simulink model "PubIfDecisionTOS_MDL"  (R2020b)
settings: configuration reference "DspaceConfig" (kept outside this file)
PostLoadFcn:
  | if any(exist('dsrtsu_mdlpostloadfcn', 'file') ~= 0), dsrtsu_mdlpostloadfcn('Execute', bdroot); end
InitFcn:
  | , if any(exist('dsmpb_private', 'file') ~= 0), dsmpb_private('dsmpb_mdlclblib', 'Init', bdroot); end,
undefined symbols (not defined in the file or in its folder): C_TOS_ACCEgoRAxletoFbumplength_m, C_TOS_ACCTargetFront_Flag, C_TOS_AEBJAPedObjDxThre_Val, C_TOS_AEBJAPedObjDyThre_Val, C_TOS_AEBJATargetSize_Val, C_TOS_AEBJAVehObjDxThre_Val, C_TOS_AEBJAVehObjDyThre_Val, C_TOS_AEBJuncPedTargetSize_Val, C_TOS_AEBLatObjDxThre_Val, C_TOS_AEBLatPedDyThre_Val, C_TOS_AEBLatTargetSize_Val, C_TOS_AEBLongTargetInEgoFront_Flag, C_TOS_axAbsGround_Parameter, C_TOS_CameraConfirmedFlag, C_TOS_CNsubjWidth, C_TOS_CurrentLaneCoreMinWidth_Val, C_TOS_CutInProb_Val_Zero, C_TOS_CutOutProb_Val_Zero, C_TOS_D2R_Val, C_TOS_DefaultValueObjectToCenterLine_dy, C_TOS_EgoCarWidth_Val, C_TOS_EgoDxRefPoint_m, C_TOS_EgoRAxletoFbumplength_m, C_TOS_HalfWidthVehicle_Con, C_TOS_HWA_CurrentLaneFlag, C_TOS_HWA_LeftLaneFlag, C_TOS_HWA_MovingDir_Vaild, C_TOS_HWA_MovState_Vaild, C_TOS_HWA_RightLaneFlag, C_TOS_LaneLineCourseErrorFront, C_TOS_LaneLineCourseErrorRear, C_TOS_MotorbikeDefaultWidth_m, C_TOS_NumberOfEffectiveTargets, C_TOS_Obj_Age_Val, C_TOS_Objdx_Constraint_Val, C_TOS_ObjectDefaultWidth_m, C_TOS_ObjInCurrentLane_Val, C_TOS_ObjInCurrentLaneValid, C_TOS_ObjInLeftLaneValid, C_TOS_ObjInRightLaneValid, C_TOS_ObjNotInCurrentLane_Val, C_TOS_ObjNotREElementType, C_TOS_ObjPredictDis_dy_ConstantVal_Zeros, C_TOS_ObjToCenterLine_ConstantVal_Zeros, C_TOS_OFMObjIDInvilad_Val, C_TOS_PIL_LatDisCons_Val_zero, C_TOS_PIL_ObjectCutInFlag_b, C_TOS_PIL_ObjectCutOutFlag_b, C_TOS_PIL_ObjLaneProb_al_Val, C_TOS_PP_ObjFusType_FC_Confirm_b, C_TOS_PP_ObjFusType_FC_FR_Confirm_b, C_TOS_PP_ObjFusType_FR_Confirm_b, C_TOS_RE_80BoolDefault_Val, C_TOS_RE_80Single181Default_Val, C_TOS_RE_80Single255Default_Val, C_TOS_RE_80Uint8Default_Val, C_TOS_RE_D2R, C_TOS_RE_D_180_Val, C_TOS_RE_InvalidObjectID_Val, C_TOS_RE_InvalidTargetChainDir_Val ... (+142)
libraries: simulink x1650, TOS_LIB x361, canfdmsglib x14
(part 26 of 69)

== system PubIfDecisionTOS_MDL/TOS_20201112/TOS_2012080320/PP1128/AAT-AdditionalAttributes/PP_SignalProcessing/PP_SignalProcessing/ObjFusTypeConfirm/ObjFusType ==
  Enumerated Constant : simulink/Sources/Enumerated Constant  OutDataTypeStr=Enum: OFM_OBJ_FUSTYPE  Value=OFM_OBJ_FUSTYPE.FC_FR  SampleTime=inf
      settings: AttributesFormatString=OFM_OBJ_FUSTYPE.FC_FR = 3
  Enumerated Constant1 : simulink/Sources/Enumerated Constant  OutDataTypeStr=Enum: OFM_OBJ_FUSTYPE  Value=OFM_OBJ_FUSTYPE.FC_FR_CL  SampleTime=inf
      settings: AttributesFormatString=OFM_OBJ_FUSTYPE.FC_FR_CL=7
  Enumerated Constant10 : simulink/Sources/Enumerated Constant  OutDataTypeStr=Enum: OFM_OBJ_FUSTYPE  Value=OFM_OBJ_FUSTYPE.FC_FR_CR_BR  SampleTime=inf
      settings: AttributesFormatString=OFM_OBJ_FUSTYPE.FC_FR_CR_BR=43
  Enumerated Constant11 : simulink/Sources/Enumerated Constant  OutDataTypeStr=Enum: OFM_OBJ_FUSTYPE  Value=OFM_OBJ_FUSTYPE.FC_FR_CL_CR_BR  SampleTime=inf
      settings: AttributesFormatString=OFM_OBJ_FUSTYPE.FC_FR_CL_CR_BR=47
  Enumerated Constant12 : simulink/Sources/Enumerated Constant  OutDataTypeStr=Enum: OFM_OBJ_FUSTYPE  Value=OFM_OBJ_FUSTYPE.FC_FR_BL_BR  SampleTime=inf
      settings: AttributesFormatString=OFM_OBJ_FUSTYPE.FC_FR_BL_BR=51
  Enumerated Constant13 : simulink/Sources/Enumerated Constant  OutDataTypeStr=Enum: OFM_OBJ_FUSTYPE  Value=OFM_OBJ_FUSTYPE.FC_FR_CR_BL_BR  SampleTime=inf
      settings: AttributesFormatString=OFM_OBJ_FUSTYPE.FC_FR_CR_BL_BR=59
  Enumerated Constant14 : simulink/Sources/Enumerated Constant  OutDataTypeStr=Enum: OFM_OBJ_FUSTYPE  Value=OFM_OBJ_FUSTYPE.FC_FR_CL_BL_BR  SampleTime=inf
      settings: AttributesFormatString=OFM_OBJ_FUSTYPE.FC_FR_CL_BL_BR=55
  Enumerated Constant15 : simulink/Sources/Enumerated Constant  OutDataTypeStr=Enum: OFM_OBJ_FUSTYPE  Value=OFM_OBJ_FUSTYPE.FC_FR_CL_CR_BL_BR  SampleTime=inf
      settings: AttributesFormatString=OFM_OBJ_FUSTYPE.FC_FR_CL_CR_BL_BR=63
  Enumerated Constant16 : simulink/Sources/Enumerated Constant  OutDataTypeStr=Enum: OFM_OBJ_FUSTYPE  Value=OFM_OBJ_FUSTYPE.FR_BL  SampleTime=inf
      settings: AttributesFormatString=OFM_OBJ_FUSTYPE.FR_BL = 18
  Enumerated Constant17 : simulink/Sources/Enumerated Constant  OutDataTypeStr=Enum: OFM_OBJ_FUSTYPE  Value=OFM_OBJ_FUSTYPE.FR_CL_CR_BL  SampleTime=inf
      settings: AttributesFormatString=OFM_OBJ_FUSTYPE.FR_CL_CR_BL = 30
  Enumerated Constant18 : simulink/Sources/Enumerated Constant  OutDataTypeStr=Enum: OFM_OBJ_FUSTYPE  Value=OFM_OBJ_FUSTYPE.FR_CR_BL_BR  SampleTime=inf
      settings: AttributesFormatString=OFM_OBJ_FUSTYPE.FR_CR_BL_BR = 58
  Enumerated Constant19 : simulink/Sources/Enumerated Constant  OutDataTypeStr=Enum: OFM_OBJ_FUSTYPE  Value=OFM_OBJ_FUSTYPE.FR_CL_BR  SampleTime=inf
      settings: AttributesFormatString=OFM_OBJ_FUSTYPE.FR_CL_BR = 38
  Enumerated Constant2 : simulink/Sources/Enumerated Constant  OutDataTypeStr=Enum: OFM_OBJ_FUSTYPE  Value=OFM_OBJ_FUSTYPE.FC_FR_CR  SampleTime=inf
      settings: AttributesFormatString=OFM_OBJ_FUSTYPE.FC_FR_CR=11
  Enumerated Constant20 : simulink/Sources/Enumerated Constant  OutDataTypeStr=Enum: OFM_OBJ_FUSTYPE  Value=OFM_OBJ_FUSTYPE.FR  SampleTime=inf
      settings: AttributesFormatString=OFM_OBJ_FUSTYPE.FR = 2
  Enumerated Constant21 : simulink/Sources/Enumerated Constant  OutDataTypeStr=Enum: OFM_OBJ_FUSTYPE  Value=OFM_OBJ_FUSTYPE.FR_CL_CR_BR  SampleTime=inf
      settings: AttributesFormatString=OFM_OBJ_FUSTYPE.FR_CL_CR_BR = 46
  Enumerated Constant22 : simulink/Sources/Enumerated Constant  OutDataTypeStr=Enum: OFM_OBJ_FUSTYPE  Value=OFM_OBJ_FUSTYPE.FR_BR  SampleTime=inf
      settings: AttributesFormatString=OFM_OBJ_FUSTYPE.FR_BR = 34
  Enumerated Constant23 : simulink/Sources/Enumerated Constant  OutDataTypeStr=Enum: OFM_OBJ_FUSTYPE  Value=OFM_OBJ_FUSTYPE.FR_CL_BL_BR  SampleTime=inf
      settings: AttributesFormatString=OFM_OBJ_FUSTYPE.FR_CL_BL_BR = 54
  Enumerated Constant24 : simulink/Sources/Enumerated Constant  OutDataTypeStr=Enum: OFM_OBJ_FUSTYPE  Value=OFM_OBJ_FUSTYPE.FR_CL_CR_BL_BR  SampleTime=inf
      settings: AttributesFormatString=OFM_OBJ_FUSTYPE.FR_CL_CR_BL_BR = 62
  Enumerated Constant25 : simulink/Sources/Enumerated Constant  OutDataTypeStr=Enum: OFM_OBJ_FUSTYPE  Value=OFM_OBJ_FUSTYPE.FR_BL_BR  SampleTime=inf
      settings: AttributesFormatString=OFM_OBJ_FUSTYPE.FR_BL_BR = 50
  Enumerated Constant26 : simulink/Sources/Enumerated Constant  OutDataTypeStr=Enum: OFM_OBJ_FUSTYPE  Value=OFM_OBJ_FUSTYPE.FR_CL  SampleTime=inf
      settings: AttributesFormatString=OFM_OBJ_FUSTYPE.FR_CL = 6
  Enumerated Constant27 : simulink/Sources/Enumerated Constant  OutDataTypeStr=Enum: OFM_OBJ_FUSTYPE  Value=OFM_OBJ_FUSTYPE.FR_CR  SampleTime=inf
      settings: AttributesFormatString=OFM_OBJ_FUSTYPE.FR_CR = 10
  Enumerated Constant28 : simulink/Sources/Enumerated Constant  OutDataTypeStr=Enum: OFM_OBJ_FUSTYPE  Value=OFM_OBJ_FUSTYPE.FR_CL_CR  SampleTime=inf
      settings: AttributesFormatString=OFM_OBJ_FUSTYPE.FR_CL_CR = 14
  Enumerated Constant29 : simulink/Sources/Enumerated Constant  OutDataTypeStr=Enum: OFM_OBJ_FUSTYPE  Value=OFM_OBJ_FUSTYPE.FR_CR_BL  SampleTime=inf
      settings: AttributesFormatString=OFM_OBJ_FUSTYPE.FR_CR_BL = 26
  Enumerated Constant3 : simulink/Sources/Enumerated Constant  OutDataTypeStr=Enum: OFM_OBJ_FUSTYPE  Value=OFM_OBJ_FUSTYPE.FC_FR_CL_CR  SampleTime=inf
      settings: AttributesFormatString=OFM_OBJ_FUSTYPE.FC_FR_CL_CR=15
  Enumerated Constant30 : simulink/Sources/Enumerated Constant  OutDataTypeStr=Enum: OFM_OBJ_FUSTYPE  Value=OFM_OBJ_FUSTYPE.FR_CL_BL  SampleTime=inf
      settings: AttributesFormatString=OFM_OBJ_FUSTYPE.FR_CL_BL = 22
  Enumerated Constant31 : simulink/Sources/Enumerated Constant  OutDataTypeStr=Enum: OFM_OBJ_FUSTYPE  Value=OFM_OBJ_FUSTYPE.FR_CR_BR  SampleTime=inf
      settings: AttributesFormatString=OFM_OBJ_FUSTYPE.FR_CR_BR = 42
  Enumerated Constant32 : simulink/Sources/Enumerated Constant  OutDataTypeStr=Enum: OFM_OBJ_FUSTYPE  Value=OFM_OBJ_FUSTYPE.CL  SampleTime=inf
      settings: AttributesFormatString=OFM_OBJ_FUSTYPE.CL = 4
  Enumerated Constant33 : simulink/Sources/Enumerated Constant  OutDataTypeStr=Enum: OFM_OBJ_FUSTYPE  Value=OFM_OBJ_FUSTYPE.CR  SampleTime=inf
      settings: AttributesFormatString=OFM_OBJ_FUSTYPE.CR = 8
  Enumerated Constant34 : simulink/Sources/Enumerated Constant  OutDataTypeStr=Enum: OFM_OBJ_FUSTYPE  Value=OFM_OBJ_FUSTYPE.CL_CR  SampleTime=inf
      settings: AttributesFormatString=OFM_OBJ_FUSTYPE.CL_CR = 12
  Enumerated Constant35 : simulink/Sources/Enumerated Constant  OutDataTypeStr=Enum: OFM_OBJ_FUSTYPE  Value=OFM_OBJ_FUSTYPE.BL  SampleTime=inf
      settings: AttributesFormatString=OFM_OBJ_FUSTYPE.BL = 16
  Enumerated Constant36 : simulink/Sources/Enumerated Constant  OutDataTypeStr=Enum: OFM_OBJ_FUSTYPE  Value=OFM_OBJ_FUSTYPE.CL_BL  SampleTime=inf
      settings: AttributesFormatString=OFM_OBJ_FUSTYPE.CL_BL=20
  Enumerated Constant37 : simulink/Sources/Enumerated Constant  OutDataTypeStr=Enum: OFM_OBJ_FUSTYPE  Value=OFM_OBJ_FUSTYPE.CR_BL  SampleTime=inf
      settings: AttributesFormatString=OFM_OBJ_FUSTYPE.CR_BL = 24
  Enumerated Constant38 : simulink/Sources/Enumerated Constant  OutDataTypeStr=Enum: OFM_OBJ_FUSTYPE  Value=OFM_OBJ_FUSTYPE.CL_CR_BL  SampleTime=inf
      settings: AttributesFormatString=OFM_OBJ_FUSTYPE.CL_CR_BL=28
  Enumerated Constant39 : simulink/Sources/Enumerated Constant  OutDataTypeStr=Enum: OFM_OBJ_FUSTYPE  Value=OFM_OBJ_FUSTYPE.BR  SampleTime=inf
      settings: AttributesFormatString=OFM_OBJ_FUSTYPE.BR = 32
  Enumerated Constant4 : simulink/Sources/Enumerated Constant  OutDataTypeStr=Enum: OFM_OBJ_FUSTYPE  Value=OFM_OBJ_FUSTYPE.FC_FR_BL  SampleTime=inf
      settings: AttributesFormatString=OFM_OBJ_FUSTYPE.FC_FR_BL=19
  Enumerated Constant40 : simulink/Sources/Enumerated Constant  OutDataTypeStr=Enum: OFM_OBJ_FUSTYPE  Value=OFM_OBJ_FUSTYPE.FC_CL  SampleTime=inf
      settings: AttributesFormatString=OFM_OBJ_FUSTYPE.FC_CL = 5
  Enumerated Constant41 : simulink/Sources/Enumerated Constant  OutDataTypeStr=Enum: OFM_OBJ_FUSTYPE  Value=OFM_OBJ_FUSTYPE.FC_CL_CR_BL  SampleTime=inf
      settings: AttributesFormatString=OFM_OBJ_FUSTYPE.FC_CL_CR_BL = 29
  Enumerated Constant42 : simulink/Sources/Enumerated Constant  OutDataTypeStr=Enum: OFM_OBJ_FUSTYPE  Value=OFM_OBJ_FUSTYPE.FC_CL_BR  SampleTime=inf
      settings: AttributesFormatString=OFM_OBJ_FUSTYPE.FC_CL_BR = 37
  Enumerated Constant43 : simulink/Sources/Enumerated Constant  OutDataTypeStr=Enum: OFM_OBJ_FUSTYPE  Value=OFM_OBJ_FUSTYPE.FC_CL_CR_BR  SampleTime=inf
      settings: AttributesFormatString=OFM_OBJ_FUSTYPE.FC_CL_CR_BR = 45
  Enumerated Constant44 : simulink/Sources/Enumerated Constant  OutDataTypeStr=Enum: OFM_OBJ_FUSTYPE  Value=OFM_OBJ_FUSTYPE.CL_BR  SampleTime=inf
      settings: AttributesFormatString=OFM_OBJ_FUSTYPE.CL_BR = 36
  Enumerated Constant45 : simulink/Sources/Enumerated Constant  OutDataTypeStr=Enum: OFM_OBJ_FUSTYPE  Value=OFM_OBJ_FUSTYPE.FC_CL_BL_BR  SampleTime=inf
      settings: AttributesFormatString=OFM_OBJ_FUSTYPE.FC_CL_BL_BR = 53
  Enumerated Constant46 : simulink/Sources/Enumerated Constant  OutDataTypeStr=Enum: OFM_OBJ_FUSTYPE  Value=OFM_OBJ_FUSTYPE.FC_CL_CR  SampleTime=inf
      settings: AttributesFormatString=OFM_OBJ_FUSTYPE.FC_CL_CR = 13
  Enumerated Constant47 : simulink/Sources/Enumerated Constant  OutDataTypeStr=Enum: OFM_OBJ_FUSTYPE  Value=OFM_OBJ_FUSTYPE.FC_CL_CR_BL_BR  SampleTime=inf
      settings: AttributesFormatString=OFM_OBJ_FUSTYPE.FC_CL_CR_BL_BR = 61
  Enumerated Constant48 : simulink/Sources/Enumerated Constant  OutDataTypeStr=Enum: OFM_OBJ_FUSTYPE  Value=OFM_OBJ_FUSTYPE.FC_CL_BL  SampleTime=inf
      settings: AttributesFormatString=OFM_OBJ_FUSTYPE.FC_CL_BL = 21
  Enumerated Constant49 : simulink/Sources/Enumerated Constant  OutDataTypeStr=Enum: OFM_OBJ_FUSTYPE  Value=OFM_OBJ_FUSTYPE.FC_CR  SampleTime=inf
      settings: AttributesFormatString=OFM_OBJ_FUSTYPE.FC_CR = 9
  Enumerated Constant5 : simulink/Sources/Enumerated Constant  OutDataTypeStr=Enum: OFM_OBJ_FUSTYPE  Value=OFM_OBJ_FUSTYPE.FC_FR_CL_BL  SampleTime=inf
      settings: AttributesFormatString=OFM_OBJ_FUSTYPE.FC_FR_CL_BL=23
  Enumerated Constant50 : simulink/Sources/Enumerated Constant  OutDataTypeStr=Enum: OFM_OBJ_FUSTYPE  Value=OFM_OBJ_FUSTYPE.FC_CR_BL_BR  SampleTime=inf
      settings: AttributesFormatString=OFM_OBJ_FUSTYPE.FC_CR_BL_BR = 57
  Enumerated Constant51 : simulink/Sources/Enumerated Constant  OutDataTypeStr=Enum: OFM_OBJ_FUSTYPE  Value=OFM_OBJ_FUSTYPE.FC_CR_BL  SampleTime=inf
      settings: AttributesFormatString=OFM_OBJ_FUSTYPE.FC_CR_BL = 25
  Enumerated Constant52 : simulink/Sources/Enumerated Constant  OutDataTypeStr=Enum: OFM_OBJ_FUSTYPE  Value=OFM_OBJ_FUSTYPE.FC_CR_BR  SampleTime=inf
      settings: AttributesFormatString=OFM_OBJ_FUSTYPE.FC_CR_BR = 41
  Enumerated Constant53 : simulink/Sources/Enumerated Constant  OutDataTypeStr=Enum: OFM_OBJ_FUSTYPE  Value=OFM_OBJ_FUSTYPE.FC  SampleTime=inf
      settings: AttributesFormatString=OFM_OBJ_FUSTYPE.FC = 1
  Enumerated Constant54 : simulink/Sources/Enumerated Constant  OutDataTypeStr=Enum: OFM_OBJ_FUSTYPE  Value=OFM_OBJ_FUSTYPE.FC_BL  SampleTime=inf
      settings: AttributesFormatString=OFM_OBJ_FUSTYPE.FC_BL = 17
  Enumerated Constant55 : simulink/Sources/Enumerated Constant  OutDataTypeStr=Enum: OFM_OBJ_FUSTYPE  Value=OFM_OBJ_FUSTYPE.CR_BR  SampleTime=inf
      settings: AttributesFormatString=OFM_OBJ_FUSTYPE.CR_BR = 40
  Enumerated Constant56 : simulink/Sources/Enumerated Constant  OutDataTypeStr=Enum: OFM_OBJ_FUSTYPE  Value=OFM_OBJ_FUSTYPE.FC_BR  SampleTime=inf
      settings: AttributesFormatString=OFM_OBJ_FUSTYPE.FC_BR = 33
  Enumerated Constant57 : simulink/Sources/Enumerated Constant  OutDataTypeStr=Enum: OFM_OBJ_FUSTYPE  Value=OFM_OBJ_FUSTYPE.FC_BL_BR  SampleTime=inf
      settings: AttributesFormatString=OFM_OBJ_FUSTYPE.FC_BL_BR = 49
  Enumerated Constant58 : simulink/Sources/Enumerated Constant  OutDataTypeStr=Enum: OFM_OBJ_FUSTYPE  Value=OFM_OBJ_FUSTYPE.CL_CR_BR  SampleTime=inf
      settings: AttributesFormatString=OFM_OBJ_FUSTYPE.CL_CR_BR = 44
  Enumerated Constant59 : simulink/Sources/Enumerated Constant  OutDataTypeStr=Enum: OFM_OBJ_FUSTYPE  Value=OFM_OBJ_FUSTYPE.BL_BR  SampleTime=inf
      settings: AttributesFormatString=OFM_OBJ_FUSTYPE.BL_BR = 48
  Enumerated Constant6 : simulink/Sources/Enumerated Constant  OutDataTypeStr=Enum: OFM_OBJ_FUSTYPE  Value=OFM_OBJ_FUSTYPE.FC_FR_CR_BL  SampleTime=inf
      settings: AttributesFormatString=OFM_OBJ_FUSTYPE.FC_FR_CR_BL=27
  Enumerated Constant60 : simulink/Sources/Enumerated Constant  OutDataTypeStr=Enum: OFM_OBJ_FUSTYPE  Value=OFM_OBJ_FUSTYPE.CL_BL_BR  SampleTime=inf
      settings: AttributesFormatString=OFM_OBJ_FUSTYPE.CL_BL_BR = 52
  Enumerated Constant61 : simulink/Sources/Enumerated Constant  OutDataTypeStr=Enum: OFM_OBJ_FUSTYPE  Value=OFM_OBJ_FUSTYPE.CR_BL_BR  SampleTime=inf
      settings: AttributesFormatString=OFM_OBJ_FUSTYPE.CR_BL_BR = 56
  Enumerated Constant62 : simulink/Sources/Enumerated Constant  OutDataTypeStr=Enum: OFM_OBJ_FUSTYPE  Value=OFM_OBJ_FUSTYPE.CL_CR_BL_BR  SampleTime=inf
      settings: AttributesFormatString=OFM_OBJ_FUSTYPE.CL_CR_BL_BR = 60
  Enumerated Constant7 : simulink/Sources/Enumerated Constant  OutDataTypeStr=Enum: OFM_OBJ_FUSTYPE  Value=OFM_OBJ_FUSTYPE.FC_FR_CL_CR_BL  SampleTime=inf
      settings: AttributesFormatString=OFM_OBJ_FUSTYPE.FC_FR_CL_CR_BL=31
  Enumerated Constant8 : simulink/Sources/Enumerated Constant  OutDataTypeStr=Enum: OFM_OBJ_FUSTYPE  Value=OFM_OBJ_FUSTYPE.FC_FR_BR  SampleTime=inf
      settings: AttributesFormatString=OFM_OBJ_FUSTYPE.FC_FR_BR=35
  Enumerated Constant9 : simulink/Sources/Enumerated Constant  OutDataTypeStr=Enum: OFM_OBJ_FUSTYPE  Value=OFM_OBJ_FUSTYPE.FC_FR_CL_BR  SampleTime=inf
      settings: AttributesFormatString=OFM_OBJ_FUSTYPE.FC_FR_CL_BR=39

== system PubIfDecisionTOS_MDL/TOS_20201112/TOS_2012080320/PP1128/AAT-AdditionalAttributes/RoadEdge/RE_2020_12_07/RoadEdge_V2/RoadEdgeElementFinalJudge ==
  note: 边界元素的最终判断及选择；
      |
      | 1/2/3号目标:
      | 3TargetTheta < 22度，1，2，3均为true
      |
      | 4号目标：
      | vxv_ego>16m/s && 3TargetTheta < 22度 && 4 TargetTheta（34_13） < 5度
      | vxv_ego<=16m/s && 3TargetTheta < 22度 && 4 TargetTheta（34_13） < 11度
      |
      | 5号目标：
      | vxv_ego>16m/s && 3TargetTheta < 22度 && 4 TargetTheta（34_13） < 5度 && 5 TargetTheta（45_24） < 5度
      | vxv_ego<=16m/s && 3TargetTheta < 22度 && 4 TargetTheta（34_13） < 5度 && 5 TargetTheta（45_24） < 11度
  RE_EgoLeftEdgeGroupChainInfor : Inport  OutDataTypeStr=uint8  BusOutputAsStruct=on
  RE_EgoRightEdgeGroupChainInfor : Inport  Port=2  OutDataTypeStr=uint8  BusOutputAsStruct=on
  RE_Target_Theta : Inport  Port=3  OutDataTypeStr=single  BusOutputAsStruct=on
  REStillObjectSortIndex : Inport  Port=4  OutDataTypeStr=uint8  BusOutputAsStruct=on
  vxvRefMs : Inport  Port=5  OutDataTypeStr=single  PortDimensions=1  BusOutputAsStruct=on
  RE_EdgeElementID_K1 : Inport  Port=6
  OFM_Signal : Inport  Port=7  BusOutputAsStruct=on
  Bus Creator : BusCreator  Inputs=7
  Bus Selector : BusSelector  OutputSignals=RE_EgoLeftEdgeGroupChainInfor.RE_EgoLeftEdgeGroupChainElementCout,RE_Target_Theta.RE_EgoLeft3TargetTheta,RE_Target_Theta.RE_EgoLeft2TargetTheta,REStillObjectSortIndex.RE_EgoLeftStationaryObjectsSortIndex,vxvRefMs,OFM_Signal.Object_DX,OFM_Signal.Object_DY,OFM_Signal.Object_ID,RE_EdgeElementID_K1
  Bus Selector1 : BusSelector  OutputSignals=RE_EgoRightEdgeGroupChainInfor.RE_EgoRightEdgeGroupChainElementCount,RE_Target_Theta.RE_EgoRight3TargetTheta,RE_Target_Theta.RE_EgoRight2TargetTheta,REStillObjectSortIndex.RE_EgoRightStationaryObjectsSortIndex,vxvRefMs,OFM_Signal.Object_DX,OFM_Signal.Object_DY,OFM_Signal.Object_ID,RE_EdgeElementID_K1
  EgoLeft_RoadEdgeElementsFinalJudge : Subsystem
  EgoRight_RoadEdgeElementsFinalJudge : Subsystem
  Goto1 : Goto  Commented=on  GotoTag=RE_EgoLeftEdgeElementFlag
  Goto4 : Goto  Commented=on  GotoTag=RE_EgoLeftStillTarget34_13_Theta_ALL
  Goto9 : Goto  Commented=on  GotoTag=RE_EdgeElementID
  Terminator{1..4} (4 alike) : Terminator
  RE_EgoLeft_EdgeElementType : Outport
  RE_EgoRight_EdgeElementType : Outport  Port=2
  RE_EgoLeft_EdgeElementID : Outport  Port=3
  RE_EgoRight_EdgeElementID : Outport  Port=4
  wires:
  RE_EgoLeftEdgeGroupChainInfor/1 -> Bus Creator/1  "RE_EgoLeftEdgeGroupChainInfor"
  RE_EgoRightEdgeGroupChainInfor/1 -> Bus Creator/2  "RE_EgoRightEdgeGroupChainInfor"
  REStillObjectSortIndex/1 -> Bus Creator/4  "REStillObjectSortIndex"
  vxvRefMs/1 -> Bus Creator/5  "vxvRefMs"
  OFM_Signal/1 -> Bus Creator/6  "OFM_Signal"
  Bus Creator/1 -> Bus Selector1/1, Bus Selector/1
  Bus Selector/1 -> EgoLeft_RoadEdgeElementsFinalJudge/1(RE_EgoLeftEdgeGroupChainElementCount)  "<RE_EgoLeftEdgeGroupChainElementCout>"
  EgoLeft_RoadEdgeElementsFinalJudge/1(RE_EgoLeftEdgeElementFlag) -> Goto1/1
  EgoRight_RoadEdgeElementsFinalJudge/1(RE_EgoRightEdgeElementFlag) -> Terminator1/1
  EgoLeft_RoadEdgeElementsFinalJudge/2(RE_EgoLeftEdgeElementType) -> RE_EgoLeft_EdgeElementType/1
  EgoRight_RoadEdgeElementsFinalJudge/2(RE_EgoRightEdgeElementType) -> RE_EgoRight_EdgeElementType/1
  RE_Target_Theta/1 -> Bus Creator/3  "RE_Target_Theta"
  Bus Selector1/7 -> EgoRight_RoadEdgeElementsFinalJudge/7(Object_Dy)  "<Object_DY>"
  Bus Selector1/4 -> EgoRight_RoadEdgeElementsFinalJudge/4(RE_EgoRight_StillObjSortIndex)  "<RE_EgoRightStationaryObjectsSortIndex>"
  Bus Selector1/8 -> EgoRight_RoadEdgeElementsFinalJudge/8(Object_ID)  "<Object_ID>"
  Bus Selector1/5 -> EgoRight_RoadEdgeElementsFinalJudge/5(vxvRefMs)  "<vxvRefMs>"
  Bus Selector1/1 -> EgoRight_RoadEdgeElementsFinalJudge/1(RE_EgoRightEdgeGroupChainElementCount)  "<RE_EgoRightEdgeGroupChainElementCount>"
  Bus Selector1/6 -> EgoRight_RoadEdgeElementsFinalJudge/6(Object_Dx)  "<Object_DX>"
  Bus Selector1/2 -> EgoRight_RoadEdgeElementsFinalJudge/2(RE_EgoRight_3TargetTheta)  "<RE_EgoRight3TargetTheta>"
  Bus Selector1/3 -> EgoRight_RoadEdgeElementsFinalJudge/3(RE_EgoRight_2TargetTheta)  "<RE_EgoRight2TargetTheta>"
  Bus Selector/3 -> EgoLeft_RoadEdgeElementsFinalJudge/3(RE_EgoLeft_2TargetTheta)  "<RE_EgoLeft2TargetTheta>"
  Bus Selector/4 -> EgoLeft_RoadEdgeElementsFinalJudge/4(RE_EgoLeft_StillObjSortIndex)  "<RE_EgoLeftStationaryObjectsSortIndex>"
  Bus Selector/5 -> EgoLeft_RoadEdgeElementsFinalJudge/5(vxvRefMs)  "<vxvRefMs>"
  Bus Selector/7 -> EgoLeft_RoadEdgeElementsFinalJudge/7(Object_Dy)  "<Object_DY>"
  Bus Selector/8 -> EgoLeft_RoadEdgeElementsFinalJudge/8(Object_ID)  "<Object_ID>"
  Bus Selector/6 -> EgoLeft_RoadEdgeElementsFinalJudge/6(Object_Dx)  "<Object_DX>"
  Bus Selector/2 -> EgoLeft_RoadEdgeElementsFinalJudge/2(RE_EgoLeft_3TargetTheta)  "<RE_EgoLeft3TargetTheta>"
  EgoLeft_RoadEdgeElementsFinalJudge/3(StillTarget34_13_Theta_ALL) -> Goto4/1  "RE_EgoLeftStillTarget34_13_Theta_ALL"
  EgoRight_RoadEdgeElementsFinalJudge/3(StillTarget34_13_Theta_ALL) -> Terminator3/1
  EgoLeft_RoadEdgeElementsFinalJudge/4(RE_EgoLeftEdgeElementID) -> Goto9/1, RE_EgoLeft_EdgeElementID/1
  EgoRight_RoadEdgeElementsFinalJudge/4(RE_EgoRightEdgeElementID) -> RE_EgoRight_EdgeElementID/1
  EgoLeft_RoadEdgeElementsFinalJudge/5(EdgeGroupChainElementCount_OFM) -> Terminator2/1
  EgoRight_RoadEdgeElementsFinalJudge/5(EdgeGroupChainElementCount_OFM) -> Terminator4/1
  RE_EdgeElementID_K1/1 -> Bus Creator/7  "RE_EdgeElementID_K1"
  Bus Selector/9 -> EgoLeft_RoadEdgeElementsFinalJudge/9(RE_EdgeElementID_K1)  "<RE_EdgeElementID_K1>"
  Bus Selector1/9 -> EgoRight_RoadEdgeElementsFinalJudge/9(RE_EdgeElementID_K1)  "<RE_EdgeElementID_K1>"

== system PubIfDecisionTOS_MDL/TOS_20201112/TOS_2012080320/PP1128/AAT-AdditionalAttributes/RoadEdge/RE_2020_12_07/RoadEdge_V2/RoadEdgeElementType ==
  RE_EgoLeft_EdgeElementType : Inport
  RE_EgoRight_EdgeElementType : Inport  Port=2
  RE_EgoLeft_EdgeElementID : Inport  Port=3
  RE_EgoRight_EdgeElementID : Inport  Port=4
  OFM_Signal : Inport  Port=5  BusOutputAsStruct=on
  Add1 : Sum
  Add2 : Sum
  Bus Selector : BusSelector  OutputSignals=Object_Age,Object_ID,Object_MovingState,Object_Fus_Type
  Chart : Stateflow chart  TreatAsAtomicUnit=on
  Data Type Conversion : DataTypeConversion  OutDataTypeStr=Enum: OFM_OBJ_MOVINGSTATE_E
  For Each Subsystem : Subsystem  TreatAsAtomicUnit=on
  For Each Subsystem1 : Subsystem  TreatAsAtomicUnit=on
  Unit Delay{,1..3} (4 alike) : UnitDelay  SampleTime=-1  HasFrameUpgradeWarning=on
  RE_EdgeElementType : Outport
  RE_EdgeElementID : Outport  Port=2
  wires:
  RE_EgoLeft_EdgeElementType/1 -> Add1/1
  RE_EgoRight_EdgeElementType/1 -> Add1/2
  Chart/2(RE_EdgeElementID) -> [REEdgeElementID], RE_EdgeElementID/1  "RE_EdgeElementID"
  Add2/1 -> For Each Subsystem/1(EdgeElementID), Unit Delay/1  "EdgeElementID"
  Unit Delay/1 -> For Each Subsystem/2(EdgeElementID_K1)  "EdgeElementID_K1"
  RE_EgoLeft_EdgeElementID/1 -> Add2/1
  RE_EgoRight_EdgeElementID/1 -> Add2/2
  Unit Delay1/1 -> For Each Subsystem1/2(EdgeElementType_K1)  "EdgeElementType_K1"
  Add1/1 -> Unit Delay1/1, For Each Subsystem1/1(EdgeElementType)  "EdgeElementType"
  Chart/1(RE_EdgeElementType) -> [REEdgeElementType], RE_EdgeElementType/1  "RE_EdgeElementType"
  For Each Subsystem1/1(RE_EdgeElementType) -> Chart/1(EdgeElementType)  "E_ElementType"
  For Each Subsystem/1(RE_EdgeElementID) -> Chart/2(EdgeElementID)  "E_ElementID"
  OFM_Signal/1 -> Bus Selector/1  "OFM_Signal"
  Bus Selector/1 -> Chart/3(Object_Age)  "<Object_Age>"
  Unit Delay2/1 -> Chart/7(RE_EdgeElementType_K1)  "EdgeElementType_K1"
  Unit Delay3/1 -> Chart/8(RE_EdgeElementID_K1)  "EdgeElementID_K1"
  [REEdgeElementType] -> Unit Delay2/1
  [REEdgeElementID] -> Unit Delay3/1
  Bus Selector/2 -> Chart/4(Object_ID)  "<Object_ID>"
  Bus Selector/3 -> Data Type Conversion/1  "<Object_MovingState>"
  Data Type Conversion/1 -> Chart/5(Object_MovingState)
  Bus Selector/4 -> Chart/6(Object_FusType)  "<Object_Fus_Type>"

== system PubIfDecisionTOS_MDL/TOS_20201112/TOS_2012080320/PP1128/AAT-AdditionalAttributes/RoadEdge/RE_2020_12_07/RoadEdge_V2/RoadEdgeGroupChain ==
  note: TargetChainPart
  note: TargetChain_ObjectDy_Average
  note: TargetChain_ObjectDx_Average
  note: 边界组链的计算判断 ；
      | 1)|dx-dx_average|< 35m
      |
      | 2)vxv_ego>16m/s&&|dy-dy_average|<10m
      | vxv_ego<=16m/s&&|dy-dy_average|<6m
  note: EdgeGroupChainFlag
  note: EdgeGroupChainStartIndex
  note: EdgeGroupChainElementNum
  note: SortIndex
  note: EdgeGroupChainIndex
  note: EdgeGroupChainElementCout
  RE_StillObjectSortIndex : Inport  BusOutputAsStruct=on
  RE_EgoLeftTargetChainInfor : Inport  Port=2  BusOutputAsStruct=on
  RE_EgoRightTargetChainInfor : Inport  Port=3  BusOutputAsStruct=on
  RE_TargetTheta : Inport  Port=4  BusOutputAsStruct=on
  OFM_Signal : Inport  Port=5  BusOutputAsStruct=on
  vxvRefMs : Inport  Port=6  BusOutputAsStruct=on
  Bus Creator : BusCreator  Inputs=6
  Bus Creator1 : BusCreator  Inputs=3
  Bus Creator2 : BusCreator  Inputs=3
  Bus Selector : BusSelector  OutputSignals=OFM_Signal.Object_DX,OFM_Signal.Object_DY,RE_StillObjectSortIndex.RE_EgoLeftStationaryObjectsSortIndex,RE_EgoLeftTargetChainInfor.RE_EgoLeftTargetChainElementNum,RE_EgoLeftTargetChainInfor.RE_EgoLeftTargetChainStartIndex,vxvRefMs,RE_EgoLeftTargetChainInfor.RE_EgoLeftTargetChainIndex
  Bus Selector1 : BusSelector  OutputSignals=OFM_Signal.Object_DX,OFM_Signal.Object_DY,RE_StillObjectSortIndex.RE_EgoRightStationaryObjectsSortIndex,RE_EgoRightTargetChainInfor.RE_EgoRightTargetChainElementNum,RE_EgoRightTargetChainInfor.RE_EgoRightTargetChainStartIndex,vxvRefMs,RE_EgoRightTargetChainInfor.RE_EgoRightTargetChainIndex
  Bus Selector2 : BusSelector  OutputSignals=RE_TargetTheta,RE_StillObjectSortIndex
  Bus Selector3 : BusSelector  OutputSignals=RE_StillObjectSortIndex.RE_EgoLeftStationaryObjectsSortIndex
  Bus Selector4 : BusSelector  OutputSignals=RE_StillObjectSortIndex.RE_EgoRightStationaryObjectsSortIndex
  Display{,1..8} (9 alike) : Display  Commented=on
  EgoLeft_RoadEdgeGroupChain : Stateflow chart  TreatAsAtomicUnit=on
  EgoLeft_RoadEdgeGroupChainInfo : Stateflow chart  TreatAsAtomicUnit=on
  EgoRight_RoadEdgeGroupChain : Stateflow chart  TreatAsAtomicUnit=on
  EgoRight_RoadEdgeGroupChainInfo : Stateflow chart  TreatAsAtomicUnit=on
  From : From  Commented=on  GotoTag=RE_EgoLeftStillObjectsSortIndex
  From10 : From  Commented=on  GotoTag=TargetChain_ObjectDx_Average
  From11 : From  Commented=on  GotoTag=TargetChain_ObjectDy_Average
  From12 : From  Commented=on  GotoTag=TargetChainPart
  From5 : From  Commented=on  GotoTag=RE_EgoLeftEdgeGroupChainElementCout
  From6 : From  Commented=on  GotoTag=RE_EgoLeftEdgeGroupChainElementNum
  From7 : From  Commented=on  GotoTag=RE_EgoLeftEdgeGroupChainStartIndex
  From8 : From  Commented=on  GotoTag=RE_EgoLeftEdgeGroupChainIndex
  From9 : From  Commented=on  GotoTag=RE_EgoLeftEdgeGroupChainFlag
  Goto10 : Goto  Commented=on  GotoTag=RE_EgoRightEdgeGroupChainElementNum
  Goto11 : Goto  Commented=on  GotoTag=TargetChain_ObjectDx_Average
  Goto12 : Goto  Commented=on  GotoTag=TargetChain_ObjectDy_Average
  Goto13 : Goto  Commented=on  GotoTag=TargetChainPart
  Goto3 : Goto  Commented=on  GotoTag=RE_EgoLeftEdgeGroupChainFlag
  Goto4 : Goto  Commented=on  GotoTag=RE_EgoLeftEdgeGroupChainElementNum
  Goto9 : Goto  Commented=on  GotoTag=RE_EgoRightEdgeGroupChainFlag
  Terminator : Terminator
  Terminator1 : Terminator
  Terminator2 : Terminator
  RE_EgoLeftEdgeGroupChainInfor : Outport
  RE_EgoRightEdgeGroupChainInfor : Outport  Port=2
  RE_Target_Theta : Outport  Port=3
  REStillObjectSortIndex : Outport  Port=4
  wires:
  RE_EgoLeftTargetChainInfor/1 -> Bus Creator/2  "RE_EgoLeftTargetChainInfor"
  RE_EgoRightTargetChainInfor/1 -> Bus Creator/3  "RE_EgoRightTargetChainInfor"
  RE_StillObjectSortIndex/1 -> [RE_EgoLeftStillObjectsSortIndex], Bus Creator/1  "RE_StillObjectSortIndex"
  Bus Creator/1 -> Bus Selector2/1, Bus Selector1/1, Bus Selector4/1, Bus Selector/1, Bus Selector3/1
  RE_TargetTheta/1 -> Bus Creator/4  "RE_TargetTheta"
  Bus Selector/4 -> EgoLeft_RoadEdgeGroupChain/4(TargetChainElementNum)  "<RE_EgoLeftTargetChainElementNum>"
  Bus Selector/2 -> EgoLeft_RoadEdgeGroupChain/2(ObjectDy)  "<Object_DY>"
  Bus Selector/1 -> EgoLeft_RoadEdgeGroupChain/1(ObjectDx)  "<Object_DX>"
  Bus Selector/5 -> EgoLeft_RoadEdgeGroupChain/5(TargetChainStartIndex)  "<RE_EgoLeftTargetChainStartIndex>"
  Bus Selector/3 -> EgoLeft_RoadEdgeGroupChain/3(RE_StillObjectSortIndex)  "<RE_EgoLeftStationaryObjectsSortIndex>"
  Bus Selector/6 -> EgoLeft_RoadEdgeGroupChain/6(Ego_Velocity)  "<vxvRefMs>"
  Bus Selector1/1 -> EgoRight_RoadEdgeGroupChain/1(ObjectDx)  "<Object_DX>"
  EgoLeft_RoadEdgeGroupChain/3(REGroupChainFlag) -> Goto3/1
  Bus Selector/7 -> EgoLeft_RoadEdgeGroupChain/7(RE_TargetChainIndex)  "<RE_EgoLeftTargetChainIndex>"
  Bus Selector1/3 -> EgoRight_RoadEdgeGroupChain/3(RE_StillObjectSortIndex)  "<RE_EgoRightStationaryObjectsSortIndex>"
  Bus Selector1/2 -> EgoRight_RoadEdgeGroupChain/2(ObjectDy)  "<Object_DY>"
  Bus Selector1/4 -> EgoRight_RoadEdgeGroupChain/4(TargetChainElementNum)  "<RE_EgoRightTargetChainElementNum>"
  Bus Selector1/5 -> EgoRight_RoadEdgeGroupChain/5(TargetChainStartIndex)  "<RE_EgoRightTargetChainStartIndex>"
  Bus Selector1/6 -> EgoRight_RoadEdgeGroupChain/6(Ego_Velocity)  "<vxvRefMs>"
  Bus Selector1/7 -> EgoRight_RoadEdgeGroupChain/7(RE_TargetChainIndex)  "<RE_EgoRightTargetChainIndex>"
  EgoLeft_RoadEdgeGroupChainInfo/2(GroupChainElementNum) -> Goto4/1  "RE_EgoLeftEdgeGroupChainElementNum"
  [RE_EgoRightEdgeGroupChainStartIndex] -> Bus Creator2/2  "RE_EgoRightEdgeGroupChainStartIndex"
  Bus Selector2/1 -> RE_Target_Theta/1  "<RE_TargetTheta>"
  Bus Selector2/2 -> REStillObjectSortIndex/1  "<RE_StillObjectSortIndex>"
  EgoLeft_RoadEdgeGroupChain/1(GroupChainElementCounter) -> [RE_EgoLeftEdgeGroupChainElementCout], EgoLeft_RoadEdgeGroupChainInfo/2(GroupChainElementCounter)
  [RE_EgoRightEdgeGroupChainElementCout] -> Bus Creator2/1  "RE_EgoRightEdgeGroupChainElementCount"
  EgoRight_RoadEdgeGroupChainInfo/1(GroupChainIndex) -> [RE_EgoRightEdgeGroupChainIndex], Bus Creator2/3  "RE_EgoRightEdgeGroupChainIndex"
  OFM_Signal/1 -> Bus Creator/5  "OFM_Signal"
  vxvRefMs/1 -> Bus Creator/6  "vxvRefMs"
  Bus Creator1/1 -> RE_EgoLeftEdgeGroupChainInfor/1
  Bus Creator2/1 -> RE_EgoRightEdgeGroupChainInfor/1
  From5/1 -> Display/1
  From9/1 -> Display3/1
  From8/1 -> Display2/1
  From/1 -> Display4/1
  From6/1 -> Display5/1
  From7/1 -> Display1/1
  EgoLeft_RoadEdgeGroupChain/2(GroupChainStartIndex) -> [RE_EgoLeftEdgeGroupChainStartIndex], EgoLeft_RoadEdgeGroupChainInfo/3(GroupChainStartIndex)
  Bus Selector3/1 -> EgoLeft_RoadEdgeGroupChainInfo/1(RE_StillObjectSortIndex)  "<RE_EgoLeftStationaryObjectsSortIndex>"
  EgoLeft_RoadEdgeGroupChainInfo/1(GroupChainIndex) -> Bus Creator1/3, [RE_EgoLeftEdgeGroupChainIndex]  "RE_EgoLeftEdgeGroupChainIndex"
  [RE_EgoLeftEdgeGroupChainElementCout] -> Bus Creator1/1  "RE_EgoLeftEdgeGroupChainElementCout"
  [RE_EgoLeftEdgeGroupChainStartIndex] -> Bus Creator1/2  "RE_EgoLeftEdgeGroupChainStartIndex"
  Bus Selector4/1 -> EgoRight_RoadEdgeGroupChainInfo/1(RE_StillObjectSortIndex)  "<RE_EgoRightStationaryObjectsSortIndex>"
  EgoRight_RoadEdgeGroupChain/2(GroupChainStartIndex) -> EgoRight_RoadEdgeGroupChainInfo/3(GroupChainStartIndex), [RE_EgoRightEdgeGroupChainStartIndex]
  EgoRight_RoadEdgeGroupChain/1(GroupChainElementCounter) -> EgoRight_RoadEdgeGroupChainInfo/2(GroupChainElementCounter), [RE_EgoRightEdgeGroupChainElementCout]
  EgoRight_RoadEdgeGroupChainInfo/2(GroupChainElementNum) -> Goto10/1  "RE_EgoRightEdgeGroupChainElementNum"
  EgoRight_RoadEdgeGroupChain/3(REGroupChainFlag) -> Goto9/1
  EgoLeft_RoadEdgeGroupChain/4(TargetChain_ObjectDx_Average) -> Goto11/1
  EgoLeft_RoadEdgeGroupChain/5(TargetChain_ObjectDy_Average) -> Goto12/1
  From10/1 -> Display6/1
  From11/1 -> Display7/1
  EgoLeft_RoadEdgeGroupChain/6(TargetChainPart) -> Goto13/1
  From12/1 -> Display8/1
  EgoRight_RoadEdgeGroupChain/4(TargetChain_ObjectDx_Average) -> Terminator/1
  EgoRight_RoadEdgeGroupChain/5(TargetChain_ObjectDy_Average) -> Terminator1/1
  EgoRight_RoadEdgeGroupChain/6(TargetChainPart) -> Terminator2/1

== system PubIfDecisionTOS_MDL/TOS_20201112/TOS_2012080320/PP1128/AAT-AdditionalAttributes/RoadEdge/RE_2020_12_07/RoadEdge_V2/SelectStationaryObjects ==
  note: 筛选符合条件目标
      | 将筛选出来的目标按Dx从小到大排序
  OFM_Signal : Inport  BusOutputAsStruct=on
  Bus Creator : BusCreator  Inputs=2
  Bus Selector1 : BusSelector  OutputSignals=Object_DX,Object_DY
  Bus Selector4 : BusSelector  OutputSignals=Object_ID,Object_Fus_Type,Object_MovingState,Object_DX,Object_DY,Object_Std_DX,Object_Std_DY,Object_ExistProb
  Constant : Constant  Value=C_TOS_RE_ObjectNum_Val
      settings: AttributesFormatString=%<Value> = 80
  MATLAB Function3 : MATLAB Function  TreatAsAtomicUnit=on
  SelectStationaryObject : Subsystem
  Unit Delay : UnitDelay  SampleTime=-1  HasFrameUpgradeWarning=on
  RE_StationaryObjectsSortIndex : Outport
  RE_StationaryObjectFlag : Outport  Port=2
  wires:
  SelectStationaryObject/1(RE_StationaryObjectFlag) -> MATLAB Function3/2(ObjectCondFlag), RE_StationaryObjectFlag/1  "RE_StationaryObjectFlag"
  OFM_Signal/1 -> Bus Selector1/1, Bus Selector4/1
  Constant/1 -> MATLAB Function3/1(Object_Num)
  Bus Selector4/1 -> SelectStationaryObject/1(Object_ID)  "<Object_ID>"
  Bus Selector4/2 -> SelectStationaryObject/2(Object_FusType)  "<Object_Fus_Type>"
  Bus Selector4/3 -> SelectStationaryObject/3(Object_MovingState)  "<Object_MovingState>"
  Bus Selector4/5 -> SelectStationaryObject/5(Object_Dy)  "<Object_DY>"
  Bus Selector4/6 -> SelectStationaryObject/6(Object_DxStd)  "<Object_Std_DX>"
  Bus Selector4/7 -> SelectStationaryObject/7(Object_DyStd)  "<Object_Std_DY>"
  Bus Selector4/4 -> SelectStationaryObject/4(Object_Dx)  "<Object_DX>"
  MATLAB Function3/1(ObjDisIndex_Left) -> Bus Creator/1  "RE_EgoLeftStationaryObjectsSortIndex"
  MATLAB Function3/2(ObjDisIndex_Right) -> Bus Creator/2  "RE_EgoRightStationaryObjectsSortIndex"
  Bus Creator/1 -> RE_StationaryObjectsSortIndex/1
  Bus Selector1/1 -> MATLAB Function3/3(Object_Dx)  "<Object_DX>"
  Bus Selector1/2 -> MATLAB Function3/4(Object_Dy)  "<Object_DY>"
  Bus Selector4/8 -> Unit Delay/1, SelectStationaryObject/8(Object_ExistProb)  "<Object_ExistProb>"
  Unit Delay/1 -> SelectStationaryObject/9(Object_ExistProb_K1)

== system PubIfDecisionTOS_MDL/TOS_20201112/TOS_2012080320/PP1128/AAT-AdditionalAttributes/RoadEdge/RE_2020_12_07/RoadEdge_V2/TargetChain ==
  note: 1、计算目标连线之间的夹角theta
      | 2、判断目标链的方向；直向/左向/右向
      | 同向/异向
      | 3、目标链组成元素的计算判断
  RE_StillObjectsSortIndex : Inport  OutDataTypeStr=uint8  BusOutputAsStruct=on
  OFM_Signal : Inport  Port=2  BusOutputAsStruct=on
  RE_EdgeElementID_K1 : Inport  Port=3
  Bus Creator : BusCreator  Inputs=3
  Bus Creator1 : BusCreator  Inputs=3
  Bus Creator2 : BusCreator  Inputs=3
  Bus Creator3 : BusCreator  Inputs=4
  Bus Selector : BusSelector  OutputSignals=RE_StillObjectsSortIndex.RE_EgoLeftStationaryObjectsSortIndex,OFM_Signal.Object_DX,OFM_Signal.Object_DY,OFM_Signal.Object_ID,RE_EdgeElementID_K1
  Bus Selector1 : BusSelector  OutputSignals=RE_StillObjectsSortIndex.RE_EgoRightStationaryObjectsSortIndex,OFM_Signal.Object_DX,OFM_Signal.Object_DY,OFM_Signal.Object_ID,RE_EdgeElementID_K1
  Bus Selector2 : BusSelector  OutputSignals=OFM_Signal,RE_StillObjectsSortIndex.RE_EgoLeftStationaryObjectsSortIndex,RE_StillObjectsSortIndex.RE_EgoRightStationaryObjectsSortIndex
  Bus Selector3 : BusSelector  OutputSignals=RE_StillObjectsSortIndex
  EgoLeftTargetChainDirection : Subsystem
  EgoRightTargetChainDirection : Subsystem
  ObjectIsTargetChainElement : Subsystem
  RE_StillObjectSortIndex : Outport
  RE_EgoLeftTargetChainInfor : Outport  Port=2
  RE_EgoRightTargetChainInfor : Outport  Port=3
  RE_TargetTheta : Outport  Port=4
  wires:
  EgoLeftTargetChainDirection/1(RE_EgoLeftTargetChainStartDirection) -> ObjectIsTargetChainElement/1(RE_EgoLeftTargetChainStartDirection)  "RE_EgoLeftTargetChainStartDirection"
  EgoRightTargetChainDirection/1(RE_EgoRightTargetChainStartDirection) -> ObjectIsTargetChainElement/8(RE_EgoRightTargetChainStartDirection)
  EgoLeftTargetChainDirection/2(RE_EgoLeftTargetChainDirection) -> ObjectIsTargetChainElement/2(RE_EgoLeftTargetChainDirection)  "RE_EgoLeftTargetChainDirection"
  EgoRightTargetChainDirection/2(RE_EgoRightTargetChainDirection) -> ObjectIsTargetChainElement/9(RE_EgoRightTargetChainDirection)
  RE_StillObjectsSortIndex/1 -> Bus Creator/1  "RE_StillObjectsSortIndex"
  OFM_Signal/1 -> Bus Creator/2  "OFM_Signal"
  Bus Creator/1 -> Bus Selector1/1, Bus Selector2/1, Bus Selector/1, Bus Selector3/1
  Bus Selector/1 -> EgoLeftTargetChainDirection/1(RE_EgoLeftStationaryObjectsSortIndex)  "<RE_EgoLeftStationaryObjectsSortIndex>"
  Bus Selector/2 -> EgoLeftTargetChainDirection/2(Object_Dx)  "<Object_DX>"
  Bus Selector2/1 -> ObjectIsTargetChainElement/5(OFM_Signal)  "<OFM_Signal>"
  Bus Selector2/2 -> ObjectIsTargetChainElement/6(RE_EgoLeftStillObjectsSortIndex)  "<RE_EgoLeftStationaryObjectsSortIndex>"
  Bus Selector2/3 -> ObjectIsTargetChainElement/7(RE_EgoRightStillObjectsSortIndex)  "<RE_EgoRightStationaryObjectsSortIndex>"
  Bus Selector/3 -> EgoLeftTargetChainDirection/3(Object_Dy)  "<Object_DY>"
  Bus Selector1/2 -> EgoRightTargetChainDirection/2(Object_Dx)  "<Object_DX>"
  Bus Selector1/1 -> EgoRightTargetChainDirection/1(RE_EgoRightStationaryObjectsSortIndex)  "<RE_EgoRightStationaryObjectsSortIndex>"
  Bus Selector1/3 -> EgoRightTargetChainDirection/3(Object_Dy)  "<Object_DY>"
  ObjectIsTargetChainElement/1(RE_EgoLeftTargetChainIndex) -> Bus Creator1/1  "RE_EgoLeftTargetChainIndex"
  ObjectIsTargetChainElement/5(RE_EgoRightTargetChainElementNum) -> Bus Creator2/2  "RE_EgoRightTargetChainElementNum"
  ObjectIsTargetChainElement/2(RE_EgoLeftTargetChainElementNum) -> Bus Creator1/2  "RE_EgoLeftTargetChainElementNum"
  ObjectIsTargetChainElement/4(RE_EgoRightTargetChainIndex) -> Bus Creator2/1  "RE_EgoRightTargetChainIndex"
  ObjectIsTargetChainElement/6(RE_EgoRightTargetChainStartIndex) -> Bus Creator2/3  "RE_EgoRightTargetChainStartIndex"
  ObjectIsTargetChainElement/3(RE_EgoLeftTargetChainStartIndex) -> Bus Creator1/3  "RE_EgoLeftTargetChainStartIndex"
  EgoLeftTargetChainDirection/3(RE_EgoLeft3TargetTheta) -> ObjectIsTargetChainElement/3(RE_EgoLeftStill3TargetTheta)  "RE_EgoLeft3TargetTheta"
  Bus Selector3/1 -> RE_StillObjectSortIndex/1  "<RE_StillObjectsSortIndex>"
  EgoRightTargetChainDirection/3(RE_EgoRight3TargetTheta) -> ObjectIsTargetChainElement/10(RE_EgoRightStill3TargetTheta)
  ObjectIsTargetChainElement/7(RE_EgoLeft3TargetTheta) -> Bus Creator3/1  "RE_EgoLeft3TargetTheta"
  ObjectIsTargetChainElement/8(RE_EgoRight3TargetTheta) -> Bus Creator3/2  "RE_EgoRight3TargetTheta"
  EgoRightTargetChainDirection/4(RE_EgoRight2TargetTheta) -> ObjectIsTargetChainElement/11(RE_EgoRightStillTarget2Theta)
  EgoLeftTargetChainDirection/4(RE_EgoLeft2TargetTheta) -> ObjectIsTargetChainElement/4(RE_EgoLeftStillTarget2Theta)  "RE_EgoLeft2TargetTheta"
  ObjectIsTargetChainElement/9(RE_EgoLeft2TargetTheta) -> Bus Creator3/3  "RE_EgoLeft2TargetTheta"
  ObjectIsTargetChainElement/10(RE_EgoRight2TargetTheta) -> Bus Creator3/4  "RE_EgoRight2TargetTheta"
  Bus Creator1/1 -> RE_EgoLeftTargetChainInfor/1
  Bus Creator2/1 -> RE_EgoRightTargetChainInfor/1
  Bus Creator3/1 -> RE_TargetTheta/1
  Bus Selector/4 -> EgoLeftTargetChainDirection/4(Object_ID)  "<Object_ID>"
  Bus Selector1/4 -> EgoRightTargetChainDirection/4(Object_ID)  "<Object_ID>"
  RE_EdgeElementID_K1/1 -> Bus Creator/3  "RE_EdgeElementID_K1"
  Bus Selector/5 -> EgoLeftTargetChainDirection/5(RE_EdgeElementID_K1)  "<RE_EdgeElementID_K1>"
  Bus Selector1/5 -> EgoRightTargetChainDirection/5(RE_EdgeElementID_K1)  "<RE_EdgeElementID_K1>"

== system PubIfDecisionTOS_MDL/TOS_20201112/TOS_2012080320/TLJ/Pro/Pro/ObjInLane/TLJ_ObjInEgoLane_1/Prob ==
  ObjectType : Inport
  PP_MovingStateSignalProcessing : Inport  Port=2
  Compare To Constant1 : simulink/Logic and Bit Operations/Compare To Constant  relop===  const=OFM_OBJ_TYPE_E.TRUCK  OutDataTypeStr=boolean
      settings: AttributesFormatString=OFM_OBJ_TYPE_E.TRUCK = 3
  Compare To Constant2 : simulink/Logic and Bit Operations/Compare To Constant  relop===  const=ObjectMovingState_E.Still  OutDataTypeStr=boolean
      settings: AttributesFormatString=ObjectMovingState_E.Still = 1
  Compare To Constant3 : simulink/Logic and Bit Operations/Compare To Constant  relop===  const=OFM_OBJ_TYPE_E.CAR  OutDataTypeStr=boolean
      settings: AttributesFormatString=OFM_OBJ_TYPE_E.CAR = 2
  Compare To Constant4 : simulink/Logic and Bit Operations/Compare To Constant  relop===  const=OFM_OBJ_TYPE_E.MOTORBIKE  OutDataTypeStr=boolean
      settings: AttributesFormatString=OFM_OBJ_TYPE_E.MOTORBIKE = 4
  Compare To Constant5 : simulink/Logic and Bit Operations/Compare To Constant  relop===  const=OFM_OBJ_TYPE_E.PEDESTRIAN  OutDataTypeStr=boolean
      settings: AttributesFormatString=OFM_OBJ_TYPE_E.PEDESTRIAN = 6
  Compare To Constant6 : simulink/Logic and Bit Operations/Compare To Constant  relop===  const=OFM_OBJ_TYPE_E.BICYCLE  OutDataTypeStr=boolean
      settings: AttributesFormatString=OFM_OBJ_TYPE_E.BICYCLE = 5
  Compare To Constant7 : simulink/Logic and Bit Operations/Compare To Constant  relop===  const=OFM_OBJ_TYPE_E.UNKNOWN_TYPE  OutDataTypeStr=boolean
      settings: AttributesFormatString=OFM_OBJ_TYPE_E.UNKNOWN_TYPE = 1
  Compare To Constant8 : simulink/Logic and Bit Operations/Compare To Constant  relop===  const=OFM_OBJ_TYPE_E.GENERAL_OBJECT  OutDataTypeStr=boolean
      settings: AttributesFormatString=OFM_OBJ_TYPE_E.GENERAL_OBJECT = 7
  Compare To Constant9 : simulink/Logic and Bit Operations/Compare To Constant  relop===  const=OFM_OBJ_TYPE_E.ANIMAL  OutDataTypeStr=boolean
      settings: AttributesFormatString=OFM_OBJ_TYPE_E.ANIMAL = 8
  Constant1 : Constant  Value=P_TOS_CurrentLane_CARProb_Val  OutDataTypeStr=single
      settings: AttributesFormatString=P_TOS_CurrentLane_CARProb_Val = 0.4
  Constant2 : Constant  Value=P_TOS_CurrentLane_PedestrianProb_Val  OutDataTypeStr=single
      settings: AttributesFormatString=P_TOS_CurrentLane_PedestrianProb_Val = 0.65
  Constant3 : Constant  Value=P_TOS_CurrentLane_BicycleProb_Val  OutDataTypeStr=single
      settings: AttributesFormatString=P_TOS_CurrentLane_BicycleProb_Val = 0.4
  Constant4 : Constant  Value=P_TOS_CurrentLane_OthertTypeProb_Val  OutDataTypeStr=single
      settings: AttributesFormatString=P_TOS_CurrentLane_OthertTypeProb_Val = 0.4
  Constant5 : Constant  Value=P_TOS_CurrentLane_OthertTypeProb_Val  OutDataTypeStr=single
      settings: AttributesFormatString=P_TOS_CurrentLane_OthertTypeProb_Val = 0.4
  Constant6 : Constant  Value=P_TOS_CurrentLane_StillObjProb_Val  OutDataTypeStr=single
      settings: AttributesFormatString=P_TOS_CurrentLane_StillObjProb_Val = 0.5
  Data Type Conversion1 : DataTypeConversion  OutDataTypeStr=Enum: OFM_OBJ_TYPE_E
  Data Type Conversion2 : DataTypeConversion  OutDataTypeStr=Enum: ObjectMovingState_E
  Logical Operator1 : Logic  Operator=OR  Inputs=3  AllPortsSameDT=off  OutDataTypeStr=boolean
  Logical Operator2 : Logic  Operator=OR  Inputs=3  AllPortsSameDT=off  OutDataTypeStr=boolean
  Switch{1..5} (5 alike) : Switch  Criteria=u2 > Threshold
  Prob : Outport
  wires:
  Compare To Constant9/1 -> Logical Operator1/3
  Compare To Constant7/1 -> Logical Operator1/1
  Compare To Constant8/1 -> Logical Operator1/2
  Compare To Constant1/1 -> Logical Operator2/2
  Compare To Constant4/1 -> Logical Operator2/3
  Compare To Constant3/1 -> Logical Operator2/1
  PP_MovingStateSignalProcessing/1 -> Data Type Conversion2/1
  Constant6/1 -> Switch5/1
  Switch5/1 -> Prob/1
  Compare To Constant2/1 -> Switch5/2
  ObjectType/1 -> Data Type Conversion1/1
  Switch1/1 -> Switch5/3
  Constant2/1 -> Switch2/1
  Compare To Constant5/1 -> Switch2/2
  Constant3/1 -> Switch3/1
  Switch4/1 -> Switch3/3
  Switch2/1 -> Switch1/3
  Constant1/1 -> Switch1/1
  Compare To Constant6/1 -> Switch3/2
  Logical Operator2/1 -> Switch1/2
  Logical Operator1/1 -> Switch4/2
  Switch3/1 -> Switch2/3
  Constant4/1 -> Switch4/1
  Constant5/1 -> Switch4/3
  Data Type Conversion1/1 -> Compare To Constant3/1, Compare To Constant1/1, Compare To Constant4/1, Compare To Constant5/1, Compare To Constant6/1, Compare To Constant7/1, Compare To Constant8/1, Compare To Constant9/1
  Data Type Conversion2/1 -> Compare To Constant2/1
